simulink model "closedzeta_bldc"  (R2018a)
settings: Solver=VariableStepAuto  StartTime=0.0  StopTime=10  RelTol=1e-3
undefined symbols (not defined in the file): sigbuilder_block
libraries: powerlib x21, simulink x8
settings Model: Creator=Big Daddy  LastModifiedBy=Big Daddy

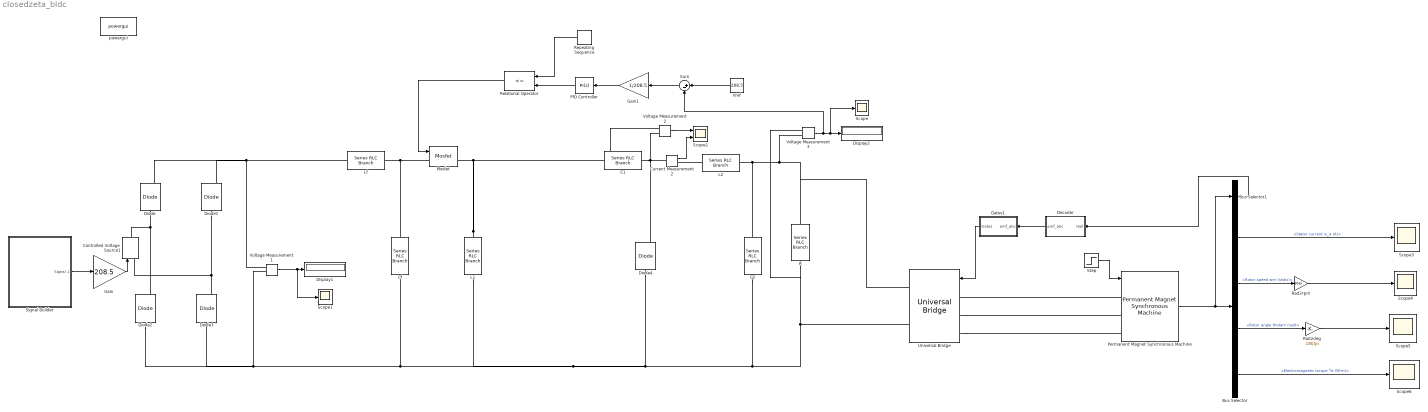
== system closedzeta_bldc ==
  Bus Selector : BusSelector  OutputSignals=Stator current is_a (A),Rotor speed wm (rad/s),Rotor angle thetam (rad),Electromagnetic torque Te (N*m)
  Bus Selector1 : BusSelector  OutputSignals=Hall effect signal h_a,Hall effect signal h_b,Hall effect signal h_c  OutputAsBus=on
  C1 : powerlib/Elements/Series RLC Branch  LConnTagsString=__new0  RConnTagsString=__new0  BranchType=C  Resistance=1  Inductance=1e-3  SetiL0=off  InitialCurrent=0  Capacitance=239e-9  Setx0=off  InitialVoltage=0  Measurements=None
  "C2 " : powerlib/Elements/Series RLC Branch  LConnTagsString=__new0  RConnTagsString=__new0  BranchType=C  Resistance=1  Inductance=1e-3  SetiL0=off  InitialCurrent=0  Capacitance=935e-6  Setx0=off  InitialVoltage=0  Measurements=None
  Cf : powerlib/Elements/Series RLC Branch  LConnTagsString=__new0  RConnTagsString=__new0  BranchType=C  Resistance=1  Inductance=1e-3  SetiL0=off  InitialCurrent=0  Capacitance=330e-9  Setx0=off  InitialVoltage=0  Measurements=None
  Controlled Voltage Source1 : powerlib/Electrical Sources/Controlled Voltage Source  Initialize=on  Source_Type=AC  Amplitude=0  Phase=0  Frequency=0  Measurements=None
  Current Measurement2 : powerlib/Measurements/Current Measurement  PhasorSimulation=off  OutputType=Complex  PSBequivalent=0
  Decoder : Subsystem
  Diode{,1..4} (5 alike) : powerlib/Power Electronics/Diode  Ron=0.001  Lon=0  Vf=0.8  IC=0  UseSnubber=0  Rs=500  Cs=250e-9  Measurements=on
  Display1 : Display
  Display2 : Display
  Gain : Gain  Gain=208.5
  Gain1 : Gain  Gain=1/208.5
  Gates1 : Subsystem
  L1 : powerlib/Elements/Series RLC Branch  LConnTagsString=__new0  RConnTagsString=__new0  BranchType=L  Resistance=1  Inductance=3.6e-3  SetiL0=off  InitialCurrent=0  Capacitance=1e-6  Setx0=off  InitialVoltage=0  Measurements=None
  L2 : powerlib/Elements/Series RLC Branch  LConnTagsString=__new0  RConnTagsString=__new0  BranchType=L  Resistance=1  Inductance=0.85e-3  SetiL0=off  InitialCurrent=0  Capacitance=1e-6  Setx0=off  InitialVoltage=0  Measurements=None
  Lf : powerlib/Elements/Series RLC Branch  LConnTagsString=__new0  RConnTagsString=__new0  BranchType=L  Resistance=1  Inductance=1e-3  SetiL0=off  InitialCurrent=0  Capacitance=1e-6  Setx0=off  InitialVoltage=0  Measurements=None
  Mosfet : powerlib/Power Electronics/Mosfet  Ron=0.1  Lon=0  Rd=0.01  Vfd=0  IC=0  Rs=1e5  Cs=inf  Measurements=on
  PID Controller : simulink/Continuous/PID Controller  Controller=PI  TimeDomain=Discrete-time  SampleTime=-1  IntegratorMethod=Forward Euler  FilterMethod=Forward Euler  Form=Parallel  UseFilter=on  ControllerParametersSource=internal  P=15  I=80  D=0  N=100  InitialConditionSource=internal  InitialConditionForIntegrator=0  InitialConditionForFilter=0  ExternalReset=none  LimitOutput=on  UpperSaturationLimit=0.9  LowerSaturationLimit=0.1  LinearizeAsGain=on  AntiWindupMode=none  Kb=1  TrackingMode=off  Kt=1  PParamMin=[]  PParamMax=[]  IParamMin=[]  IParamMax=[]  DParamMin=[]  DParamMax=[]  NParamMin=[]  NParamMax=[]  KbParamMin=[]  KbParamMax=[]  KtParamMin=[]  KtParamMax=[]  POutMin=[]  POutMax=[]  IOutMin=[]  IOutMax=[]  DOutMin=[]  DOutMax=[]  NOutMin=[]  NOutMax=[]  KbOutMin=[]  KbOutMax=[]  KtOutMin=[]  KtOutMax=[]  IntegratorOutMin=[]  IntegratorOutMax=[]  FilterOutMin=[]  FilterOutMax=[]  SumOutMin=[]  SumOutMax=[]  SumI1OutMin=[]  SumI1OutMax=[]  SumI2OutMin=[]  SumI2OutMax=[]  SumI3OutMin=[]  SumI3OutMax=[]  SumDOutMin=[]  SumDOutMax=[]  SaturationOutMin=[]  SaturationOutMax=[]  IntegratorContinuousStateAttributes=''  IntegratorStateMustResolveToSignalObject=off  IntegratorRTWStateStorageClass=Auto  FilterContinuousStateAttributes=''  FilterStateMustResolveToSignalObject=off  FilterRTWStateStorageClass=Auto  DifferentiatorICPrevScaledInput=0  DifferentiatorOutMin=[]  DifferentiatorOutMax=[]  FilterDiffOutCoefMin=[]  FilterDiffOutCoefMax=[]  SumDenOutMin=[]  SumDenOutMax=[]  SumNumOutMin=[]  SumNumOutMax=[]  ReciprocalOutMin=[]  ReciprocalOutMax=[]  DivideOutMin=[]  DivideOutMax=[]  TunerSelectOption=Transfer Function Based (PID Tuner App)
  Permanent Magnet Synchronous Machine : powerlib/Machines/Permanent Magnet Synchronous Machine  NbPhases=3  FluxDistribution=Trapezoidal  RotorType=Round  MechanicalLoad=Torque Tm  PresetModel=No  ShowDetailedParameters=on  MeasurementBus=off  Resistance=2.875  Inductance=8.5e-3  dqInductances=[8.5e-3, 8.5e-3]  La=0.000835  MachineConstant=Flux linkage established by magnets (V.s)  Flux=0.175  VoltageCst=146.6077  TorqueCst=1.4  Flat=120  Mechanical=[ 0.8e-3, 1e-3 4]  PolePairs=4  InitialConditions=[0,0, 0,0]  InitialConditions5ph=[0 0 0 0 0 0]  TsPowergui=0  TsBlock=-1  RefAngle=90 degrees behind phase A axis (modified Park)
      settings: SourceProductName=Simscape Power Systems
  R : powerlib/Elements/Series RLC Branch  LConnTagsString=__new0  RConnTagsString=__new0  BranchType=R  Resistance=400  Inductance=1e-3  SetiL0=off  InitialCurrent=0  Capacitance=1e-6  Setx0=off  InitialVoltage=0  Measurements=None
  Rad2deg : Gain  Gain=180/pi
  Rad2rpm : Gain  Gain=30/pi
  Relational Operator : RelationalOperator  Operator=<=  OutDataTypeStr=boolean  RndMeth=Simplest
  Repeating Sequence : simulink/Sources/Repeating Sequence  rep_seq_t=[0 .0002]  rep_seq_y=[0 1]
  Scope{,1,3..6} (6 alike) : Scope
  Scope2 : Scope  NumInputPorts=2
  Signal Builder : Subsystem  Tag=STV Subsys  LoadFcn=sigbuilder_block('load');  StartFcn=sigbuilder_block('start');  StopFcn=sigbuilder_block('stop');  ClipboardFcn=sigbuilder_block('clipboard');  mask(Sigbuilder block){tuvar=[0:10]}
      mask help: Simulink:masks:SigbuilderBlock_MD
      mask init:
      | if ~strcmp(get_param(bdroot(gcbh),'SimulationStatus'),'stopped') tuvar = sigbuilder_block('maskInit'); end
      settings: CopyFcn=sigbuilder_block('copy');  DeleteFcn=sigbuilder_block('delete');  ModelCloseFcn=sigbuilder_block('modelClose');  PreSaveFcn=sigbuilder_block('preSave');  PauseFcn=sigbuilder_block('pause');  ContinueFcn=sigbuilder_block('continue');  NameChangeFcn=sigbuilder_block('namechange');  OpenFcn=sigbuilder_block('open',[437.6 199.2 550.4 400 ]);  CloseFcn=sigbuilder_block('close');
      mask Display: plot(0, 0, 100, 100,[2, 2, 32, 32, 2], [68, 8, 8, 68, 68],[32, 2], [38, 38], [32, 19, 2],[53, 60, 44], [32, 17, 17, 2],[16, 16, 31, 31]);txt = getActiveGroup(gcbh);text(2, 100, txt,'verticalAlignment', 'top');
  Step : Step  Time=0  After=0.1  SampleTime=5e-6
  Sum : Sum  Inputs=|+-
  Universal Bridge : powerlib/Power Electronics/Universal Bridge  Arms=3  SnubberResistance=1e5  SnubberCapacitance=inf  Device=MOSFET / Diodes  Ron=1e-3  Lon=0  ForwardVoltages="[  0  0  ]"  ForwardVoltage=0  GTOparameters=[ 10e-6 , 20e-6 ]  IGBTparameters=[ 1e-6 , 2e-6 ]  Measurements=None  Measurements_2=None  converterType=Rectifier
  Voltage Measurement1 : powerlib/Measurements/Voltage Measurement  PhasorSimulation=off  OutputType=Complex  PSBequivalent=0
  Voltage Measurement2 : powerlib/Measurements/Voltage Measurement  PhasorSimulation=off  OutputType=Complex  PSBequivalent=0
  Voltage Measurement3 : powerlib/Measurements/Voltage Measurement  PhasorSimulation=off  OutputType=Complex  PSBequivalent=0
  Vref : Constant  Value=208.5
  powergui : powerlib/powergui  Priority=1  SimulationMode=Discrete  SampleTime=5e-6  frequency=50  Iterations=50  frequencyindice=0  Pbase=100e6  ErrMax=1e-4  UnitsV=kV  UnitsW=MW  buscounter=0  FunctionMessages=off  echomessages=off  EnableUseOfTLC=off  CurrentSourceSwitches=off  DisableSnubberDevices=off  DisableRonSwitches=off  DisableVfSwitches=off  DisplayEquations=off  SolverType=Tustin/Backward Euler (TBE)  Interpol=off  ExternalGateDelay=off  methode=off  Ts=100  x0status=blocks  SPID=on  SwTol=0  HookPort=off  RestoreLinks=warning  ResistiveCurrentMeasurement=off  Frange=[0:2:500]  Ylog=off  Xlog=on  ShowGrid=off  save=off  variable=ZData  structure=0  ZoomFFT=off  StartTime=0.0  cycles=1  DisplayStyle=1  fundamental=60  FreqAxis=off  MaxFrequency=1000  frequencyindicesteady=1  RmsSteady=1  display=off
  wires:
  Relational Operator/1 -> Mosfet/1
  Decoder/1(emf_abc) -> Gates1/1("emf_abc ")
  Bus Selector1/1 -> Decoder/1("Hall ")
  Current Measurement2/1 -> Scope2/2
  Bus Selector/2 -> Rad2rpm/1  "<Rotor speed wm (rad/s)>"
  Step/1 -> Permanent Magnet Synchronous Machine/1
  Bus Selector/3 -> Rad2deg/1  "<Rotor angle thetam (rad)>"
  Bus Selector/1 -> Scope3/1  "<Stator current is_a (A)>"
  Voltage Measurement2/1 -> Scope2/1
  Permanent Magnet Synchronous Machine/1 -> Bus Selector1/1, Bus Selector/1
  Signal Builder/1(Signal 1) -> Gain/1
  Gates1/1(Gates) -> Universal Bridge/1
  Rad2rpm/1 -> Scope4/1
  Rad2deg/1 -> Scope5/1
  Gain/1 -> Controlled Voltage Source1/1
  Bus Selector/4 -> Scope6/1  "<Electromagnetic torque Te (N*m)>"
  Voltage Measurement1/1 -> Scope1/1, Display1/1
  Repeating Sequence/1 -> Relational Operator/1
  Sum/1 -> Gain1/1
  Gain1/1 -> PID Controller/1
  Vref/1 -> Sum/1
  PID Controller/1 -> Relational Operator/2
  Voltage Measurement3/1 -> Sum/2, Scope/1, Display2/1
  connections:
  "C2 "/LConn1 -- Diode3/LConn1 -- Diode2/LConn1 -- Voltage Measurement1/LConn2 -- Cf/LConn1 -- L1/LConn1 -- Diode4/LConn1 -- Universal Bridge/RConn2 -- R/LConn1 -- Voltage Measurement3/LConn2
  L1/RConn1 -- Mosfet/RConn1 -- Voltage Measurement2/LConn1 -- C1/LConn1
  Diode/RConn1 -- Diode1/RConn1 -- Voltage Measurement1/LConn1 -- Lf/LConn1
  Voltage Measurement3/LConn1 -- Universal Bridge/RConn1 -- R/RConn1 -- "C2 "/RConn1 -- L2/RConn1
  Diode2/RConn1 -- Controlled Voltage Source1/RConn1 -- Diode/LConn1
  Cf/RConn1 -- Lf/RConn1 -- Mosfet/LConn1
  Voltage Measurement2/LConn2 -- Diode4/RConn1 -- Current Measurement2/LConn1 -- C1/RConn1
  Diode1/LConn1 -- Controlled Voltage Source1/LConn1 -- Diode3/RConn1
  Permanent Magnet Synchronous Machine/LConn1 -- Universal Bridge/LConn1
  L2/LConn1 -- Current Measurement2/RConn1
  Universal Bridge/LConn2 -- Permanent Magnet Synchronous Machine/LConn2
  Universal Bridge/LConn3 -- Permanent Magnet Synchronous Machine/LConn3

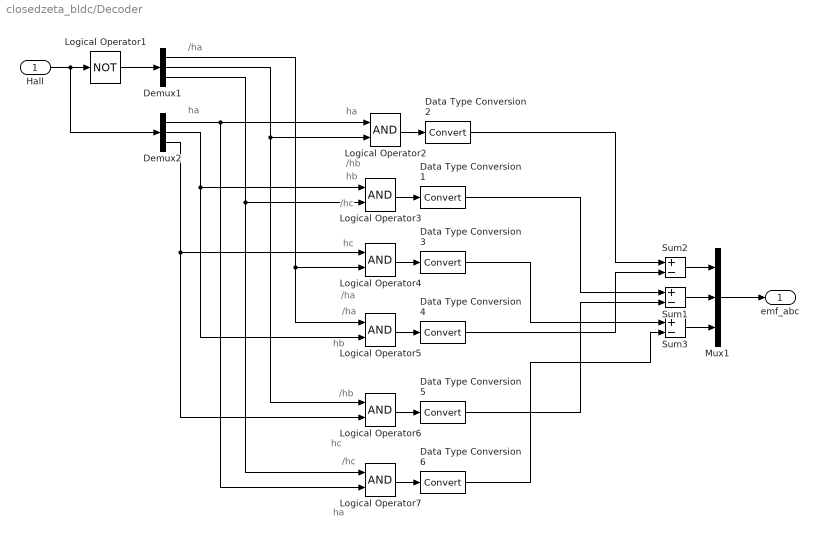
== system closedzeta_bldc/Decoder ==
  note: /ha
  note: ha
  note: ha
  note: /hb
  note: hb
  note: /hc
  note: hc
  note: /ha
  note: /ha
  note: hb
  note: /hb
  note: hc
  note: /hc
  note: ha
  "Hall " : Inport
  Data Type Conversion{1..6} (6 alike) : DataTypeConversion
  Demux1 : Demux  Outputs=3
  Demux2 : Demux  Outputs=3
  Logical Operator1 : Logic  Operator=NOT  AllPortsSameDT=off  OutDataTypeStr=boolean
  Logical Operator{2..7} (6 alike) : Logic  AllPortsSameDT=off  OutDataTypeStr=boolean
  Mux1 : Mux  Inputs=3
  Sum1 : Sum  Inputs=+-  OutDataTypeStr=double
  Sum2 : Sum  Inputs=+-  OutDataTypeStr=double
  Sum3 : Sum  Inputs=+-  OutDataTypeStr=double
  emf_abc : Outport
  wires:
  "Hall "/1 -> Logical Operator1/1, Demux2/1
  Logical Operator1/1 -> Demux1/1
  Demux2/3 -> Logical Operator4/1, Logical Operator6/2
  Demux2/2 -> Logical Operator3/1, Logical Operator5/2
  Demux2/1 -> Logical Operator2/1, Logical Operator7/2
  Demux1/3 -> Logical Operator3/2, Logical Operator7/1
  Demux1/2 -> Logical Operator2/2, Logical Operator6/1
  Demux1/1 -> Logical Operator4/2, Logical Operator5/1
  Logical Operator2/1 -> Data Type Conversion2/1
  Sum2/1 -> Mux1/1
  Sum1/1 -> Mux1/2
  Sum3/1 -> Mux1/3
  Mux1/1 -> emf_abc/1
  Logical Operator3/1 -> Data Type Conversion1/1
  Logical Operator4/1 -> Data Type Conversion3/1
  Logical Operator5/1 -> Data Type Conversion4/1
  Logical Operator6/1 -> Data Type Conversion5/1
  Logical Operator7/1 -> Data Type Conversion6/1
  Data Type Conversion2/1 -> Sum2/1
  Data Type Conversion4/1 -> Sum2/2
  Data Type Conversion1/1 -> Sum1/1
  Data Type Conversion5/1 -> Sum1/2
  Data Type Conversion3/1 -> Sum3/1
  Data Type Conversion6/1 -> Sum3/2

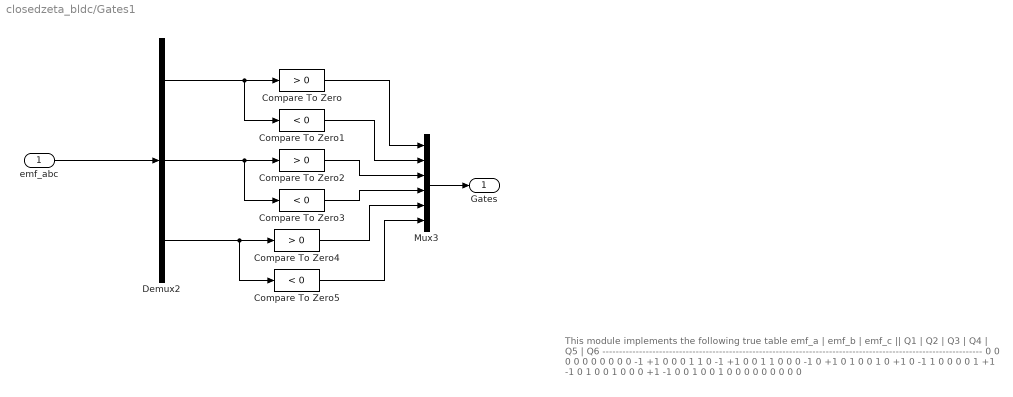
== system closedzeta_bldc/Gates1 ==
  note: This module implements the following true table
      |
      |    emf_a   |   emf_b   |   emf_c   ||   Q1   |   Q2   |   Q3   |   Q4   |   Q5   |   Q6
      |     ------------------------------------------------------------------------------------------------------------------
      |       0              0                0            0          0          0           0        0        0
      |       0               -1              +1          0          0          0           1        1        0
      |     -1              +1                0          0          1          1           0        0        0
      |     -1               0               +1          0          1         0           0        1        0
      |    +1               0                -1          1          0          0           0        0        1
      |    +1              -1                0           1          0          0           1        0        0
      |      0              +1               -1           0          0          1           0        0        1
      |     0              0                0             0          0          0           0        0        0
  "emf_abc " : Inport
  Compare To Zero : simulink/Logic and Bit Operations/Compare To Zero  relop=>  OutDataTypeStr=boolean  ZeroCross=off
  Compare To Zero1 : simulink/Logic and Bit Operations/Compare To Zero  relop=<  OutDataTypeStr=boolean  ZeroCross=off
  Compare To Zero2 : simulink/Logic and Bit Operations/Compare To Zero  relop=>  OutDataTypeStr=boolean  ZeroCross=off
  Compare To Zero3 : simulink/Logic and Bit Operations/Compare To Zero  relop=<  OutDataTypeStr=boolean  ZeroCross=off
  Compare To Zero4 : simulink/Logic and Bit Operations/Compare To Zero  relop=>  OutDataTypeStr=boolean  ZeroCross=off
  Compare To Zero5 : simulink/Logic and Bit Operations/Compare To Zero  relop=<  OutDataTypeStr=boolean  ZeroCross=off
  Demux2 : Demux  Outputs=3
  Mux3 : Mux  Inputs=6
  Gates : Outport
  wires:
  "emf_abc "/1 -> Demux2/1
  Mux3/1 -> Gates/1
  Demux2/1 -> Compare To Zero/1, Compare To Zero1/1
  Demux2/2 -> Compare To Zero2/1, Compare To Zero3/1
  Demux2/3 -> Compare To Zero4/1, Compare To Zero5/1
  Compare To Zero/1 -> Mux3/1
  Compare To Zero1/1 -> Mux3/2
  Compare To Zero2/1 -> Mux3/3
  Compare To Zero3/1 -> Mux3/4
  Compare To Zero4/1 -> Mux3/5
  Compare To Zero5/1 -> Mux3/6

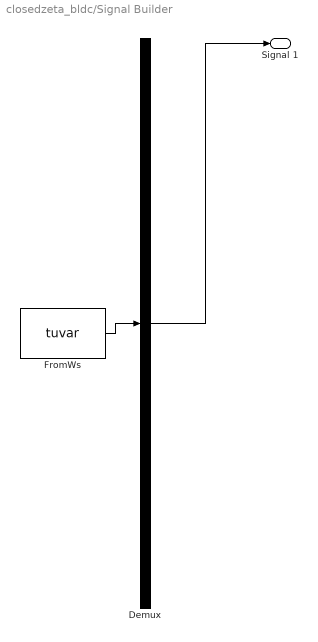
== system closedzeta_bldc/Signal Builder ==
  Demux : Demux  Tag=STV Demux  Outputs=1
  FromWs : FromWorkspace  Tag=STV FromWs  VariableName=tuvar  SampleTime=0
      SigBuilderData=|
      | common.afterFinalStr = 'Extrapolate'
      | common.sampleTime = 0
      | dataSet.timeRange = [0 10]
      | dataSet.name = 'Group 1'
      | sbobj.Groups.Name = 'Group 1'
      | sbobj.Groups.Signals.Name = 'Signal 1'
      | sbobj.Groups.Signals.XData = [0 1 2 3 10]
      | sbobj.Groups.Signals.YData = [0.65 0.65 0.65 0.65 0.65]
  Signal 1 : Outport  Tag=STV Outport
  wires:
  Demux/1 -> Signal 1/1
  FromWs/1 -> Demux/1
